simulink model "FFR_3area_2"  (R2015a)
settings: Solver=ode45  StartTime=0.0  StopTime=100  RelTol=1e-3
values from neighbouring files (symbols this model uses):
  beta = [0.3483 0.3827 0.3692]    [init_FFR_3area.m]    (also in init_FFR_3area_2.m; init_FFR_3area_3.m; init_FFR_3area_4.m; init_FFR_3area_5.m)
  D = 0.015    [init_FFR_1_0.m]    (also in init_FFR_1_1.m; init_FFR_3area.m = [0.015 0.016 0.015]; init_FFR_3area_2.m = [0.015 0.016 0.015]; init_FFR_3area_3.m = [0.015 0.016 0.015])
  H = 0.0833    [init_FFR_1_0.m]    (also in init_FFR_1_1.m; init_FFR_3area.m = [0.1667 0.2017 0.1247] .* 0.5; init_FFR_3area_2.m = [0.1667 0.2017 0.1247] .* 0.5; init_FFR_3area_3.m = [0.1667 0.2017 0.1247] .* 0.5)
  Ki = -0.3    [init_FFR_1_0.m]    (also in init_FFR_1_1.m = -2; init_FFR_3area.m = [-0.3 -0.2 -0.4]; init_FFR_3area_2.m = [-0.3 -0.2 -0.4]; init_FFR_3area_3.m = [-0.3 -0.2 -0.4])
  R = 3    [init_FFR_1_0.m]    (also in init_FFR_1_1.m; init_FFR_3area.m = [3 2.73 2.82]; init_FFR_3area_2.m = [3 2.73 2.82]; init_FFR_3area_3.m = [3 2.73 2.82])
  T_12 = 0.20    (= 0.2)    [allocateProduction.m]    (also in allocation.m; init_FFR_3area.m; init_FFR_3area_2.m; init_FFR_3area_3.m)
  T_13 = 0.25    [allocateProduction.m]    (also in allocation.m; init_FFR_3area.m; init_FFR_3area_2.m; init_FFR_3area_3.m)
  T_21 = 0.20    (= 0.2)    [allocateProduction.m]    (also in allocation.m; init_FFR_3area.m; init_FFR_3area_2.m; init_FFR_3area_3.m)
  T_23 = 0.12    [allocateProduction.m]    (also in allocation.m; init_FFR_3area.m; init_FFR_3area_2.m; init_FFR_3area_3.m)
  T_31 = 0.25    [allocateProduction.m]    (also in allocation.m; init_FFR_3area.m; init_FFR_3area_2.m; init_FFR_3area_3.m)
  T_32 = 0.12    [allocateProduction.m]    (also in allocation.m; init_FFR_3area.m; init_FFR_3area_2.m; init_FFR_3area_3.m)
  T_g = 0.08    [init_FFR_1_0.m]    (also in init_FFR_1_1.m; init_FFR_3area.m = [0.08 0.06 0.07]; init_FFR_3area_2.m = [0.08 0.06 0.07]; init_FFR_3area_3.m = [0.08 0.06 0.07])
  T_t = 0.40    (= 0.4)    [init_FFR_1_0.m]    (also in init_FFR_1_1.m; init_FFR_3area.m = [0.40 0.44 0.30]; init_FFR_3area_2.m = [0.40 0.44 0.30]; init_FFR_3area_3.m = [0.40 0.44 0.30])
libraries: simulink x3, aerolibanimutils x1
settings Model: Creator=tarje  LastModifiedBy=tarje

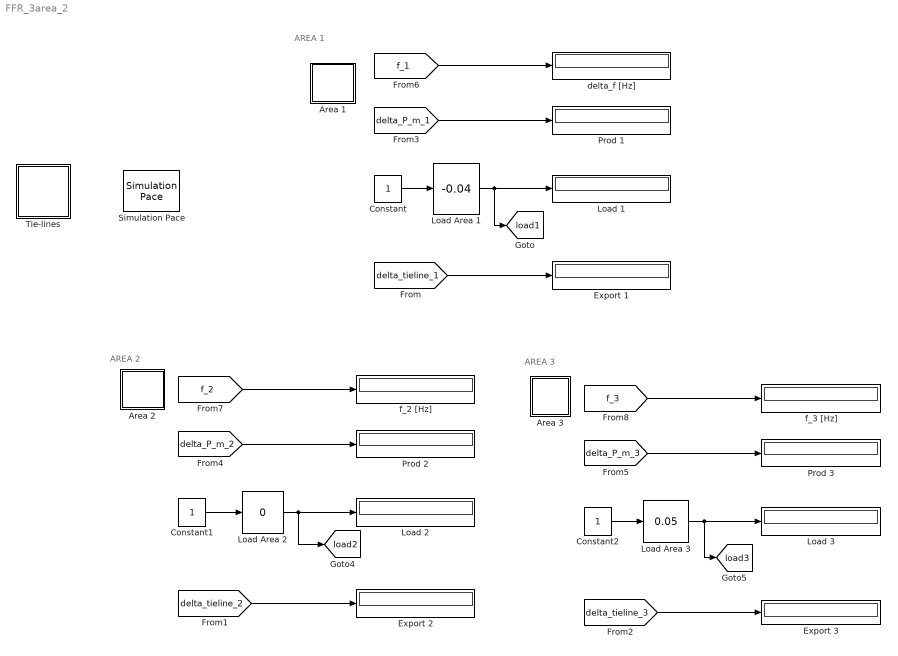
== system FFR_3area_2 ==
  note: AREA 3
  note: AREA 2
  note: AREA 1
  Area 1 : Subsystem
  Area 2 : Subsystem
  Area 3 : Subsystem
  Constant : Constant
  Constant1 : Constant
  Constant2 : Constant
  Export 1 : Display
  Export 2 : Display
  Export 3 : Display
  Load 1 : Display
  Load 2 : Display
  Load 3 : Display
  Load Area 1 : simulink/Math Operations/Slider Gain  low=-0.2  gain=-0.04  high=0.2
  Load Area 2 : simulink/Math Operations/Slider Gain  low=-0.05  gain=0  high=1
  Load Area 3 : simulink/Math Operations/Slider Gain  low=-0.05  gain=0.05  high=0.05
  Prod 1 : Display
  Prod 2 : Display
  Prod 3 : Display
  Simulation Pace : aerolibanimutils/Simulation Pace  SimulationPace=1  SleepMode=MATLAB Thread  OutputPaceError=off  SampleTime=1/30
      settings: AttributesFormatString=%<SimulationPace> sec/sec
  Tie-lines : Subsystem
  delta_f [Hz] : Display
  f_2 [Hz] : Display
  f_3 [Hz] : Display
  tag scope: load1=global, load2=global, load3=global
  wires:
  [f_1] -> delta_f [Hz]/1
  [delta_P_m_1] -> Prod 1/1
  Constant/1 -> Load Area 1/1
  Load Area 1/1 -> [load1], Load 1/1
  [f_2] -> f_2 [Hz]/1
  [delta_P_m_2] -> Prod 2/1
  Constant1/1 -> Load Area 2/1
  Load Area 2/1 -> [load2], Load 2/1
  [f_3] -> f_3 [Hz]/1
  [delta_P_m_3] -> Prod 3/1
  Constant2/1 -> Load Area 3/1
  Load Area 3/1 -> [load3], Load 3/1
  [delta_tieline_1] -> Export 1/1
  [delta_tieline_2] -> Export 2/1
  [delta_tieline_3] -> Export 3/1

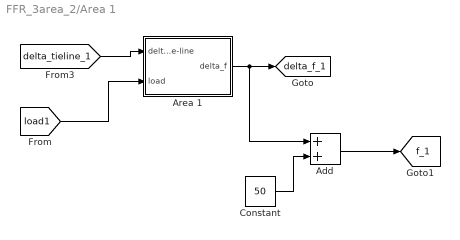
== system FFR_3area_2/Area 1 ==
  Add : Sum
  Area 1 : Subsystem
  Constant : Constant  Value=50
  tag scope: delta_f_1=global, f_1=global
  wires:
  [delta_tieline_1] -> Area 1/1(delta_tie-line)
  Area 1/1(delta_f) -> Add/1, [delta_f_1]
  [load1] -> Area 1/2(load)
  Constant/1 -> Add/2
  Add/1 -> [f_1]

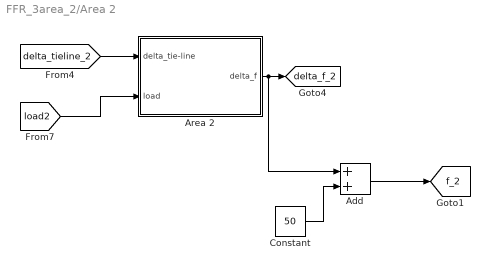
== system FFR_3area_2/Area 2 ==
  Add : Sum
  Area 2 : Subsystem
  Constant : Constant  Value=50
  tag scope: delta_f_2=global, f_2=global
  wires:
  Area 2/1(delta_f) -> Add/1, [delta_f_2]
  [load2] -> Area 2/2(load)
  [delta_tieline_2] -> Area 2/1(delta_tie-line)
  Constant/1 -> Add/2
  Add/1 -> [f_2]

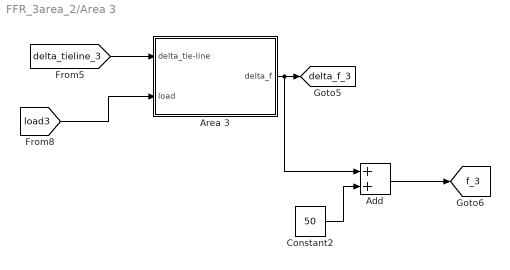
== system FFR_3area_2/Area 3 ==
  Add : Sum
  Area 3 : Subsystem
  Constant2 : Constant  Value=50
  tag scope: delta_f_3=global, f_3=global
  wires:
  [load3] -> Area 3/2(load)
  Area 3/1(delta_f) -> Add/1, [delta_f_3]
  [delta_tieline_3] -> Area 3/1(delta_tie-line)
  Add/1 -> [f_3]
  Constant2/1 -> Add/2

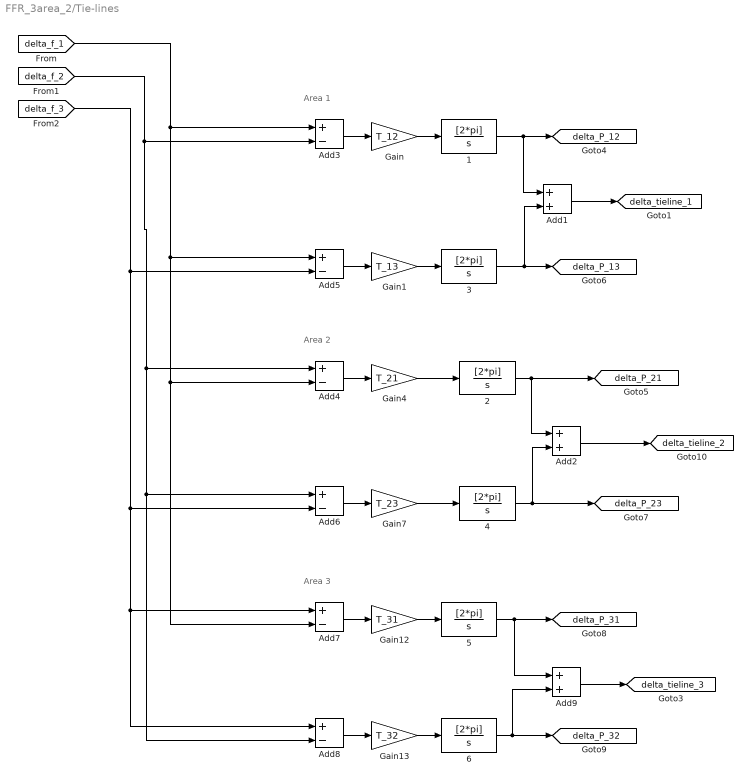
== system FFR_3area_2/Tie-lines ==
  note: Area 3
  note: Area 2
  note: Area 1
   {1..6} (6 alike) : TransferFcn  Numerator=[2*pi]  Denominator=[1 0]
  Add1 : Sum
  Add2 : Sum
  Add{3..8} (6 alike) : Sum  Inputs=+-
  Add9 : Sum
  Gain : Gain  Gain=T_12
  Gain1 : Gain  Gain=T_13
  Gain12 : Gain  Gain=T_31
  Gain13 : Gain  Gain=T_32
  Gain4 : Gain  Gain=T_21
  Gain7 : Gain  Gain=T_23
  tag scope: delta_P_12=global, delta_P_13=global, delta_P_21=global, delta_P_23=global, delta_P_31=global, delta_P_32=global, delta_tieline_1=global, delta_tieline_2=global, delta_tieline_3=global
  wires:
  [delta_f_2] -> Add3/2, Add8/2, Add6/1, Add4/1
  [delta_f_1] -> Add3/1, Add5/1, Add7/2, Add4/2
  [delta_f_3] -> Add5/2, Add8/1, Add7/1, Add6/2
  " 1"/1 -> Add1/1, [delta_P_12]
  Add3/1 -> Gain/1
  " 2"/1 -> Add2/1, [delta_P_21]
  Add4/1 -> Gain4/1
  " 3"/1 -> Add1/2, [delta_P_13]
  Add5/1 -> Gain1/1
  " 4"/1 -> Add2/2, [delta_P_23]
  Add6/1 -> Gain7/1
  " 5"/1 -> Add9/1, [delta_P_31]
  Add7/1 -> Gain12/1
  " 6"/1 -> Add9/2, [delta_P_32]
  Add8/1 -> Gain13/1
  Add9/1 -> [delta_tieline_3]
  Gain12/1 -> " 5"/1
  Gain13/1 -> " 6"/1
  Add2/1 -> [delta_tieline_2]
  Gain4/1 -> " 2"/1
  Gain7/1 -> " 4"/1
  Add1/1 -> [delta_tieline_1]
  Gain/1 -> " 1"/1
  Gain1/1 -> " 3"/1

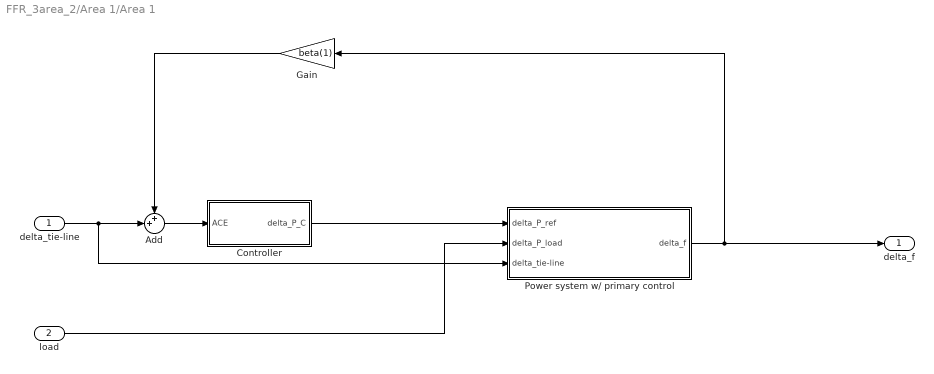
== system FFR_3area_2/Area 1/Area 1 ==
  delta_tie-line : Inport
  load : Inport  Port=2
  Add : Sum  Inputs=++|
  Controller : Subsystem
  Gain : Gain  Gain=beta(1)
  Power system w/ primary control : Subsystem
  delta_f : Outport
  wires:
  Controller/1(delta_P_C) -> Power system w/ primary control/1(delta_P_ref)
  Power system w/ primary control/1(delta_f) -> Gain/1, delta_f/1
  Gain/1 -> Add/1
  delta_tie-line/1 -> Power system w/ primary control/3(delta_tie-line), Add/2
  Add/1 -> Controller/1(ACE)
  load/1 -> Power system w/ primary control/2(delta_P_load)

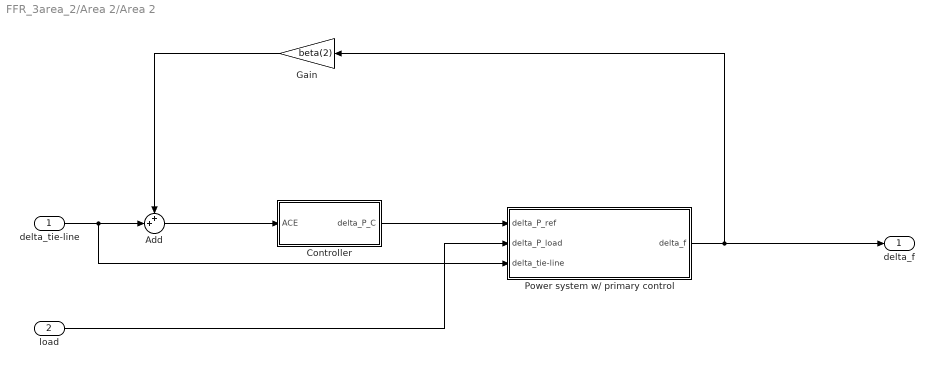
== system FFR_3area_2/Area 2/Area 2 ==
  delta_tie-line : Inport
  load : Inport  Port=2
  Add : Sum  Inputs=++|
  Controller : Subsystem
  Gain : Gain  Gain=beta(2)
  Power system w/ primary control : Subsystem
  delta_f : Outport
  wires:
  Controller/1(delta_P_C) -> Power system w/ primary control/1(delta_P_ref)
  Power system w/ primary control/1(delta_f) -> Gain/1, delta_f/1
  Gain/1 -> Add/1
  delta_tie-line/1 -> Power system w/ primary control/3(delta_tie-line), Add/2
  Add/1 -> Controller/1(ACE)
  load/1 -> Power system w/ primary control/2(delta_P_load)

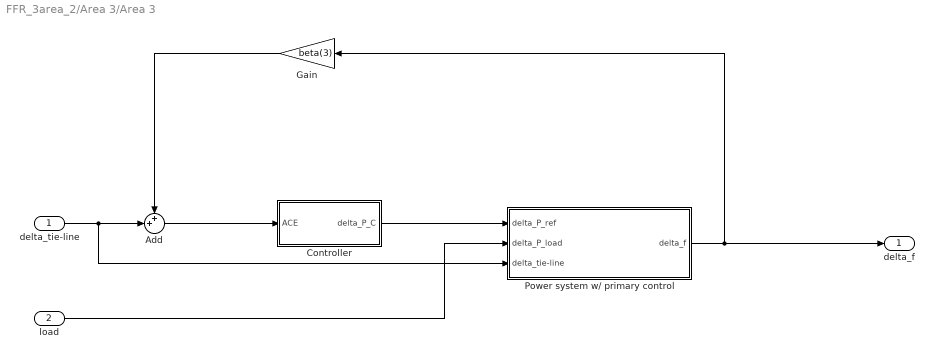
== system FFR_3area_2/Area 3/Area 3 ==
  delta_tie-line : Inport
  load : Inport  Port=2
  Add : Sum  Inputs=++|
  Controller : Subsystem
  Gain : Gain  Gain=beta(3)
  Power system w/ primary control : Subsystem
  delta_f : Outport
  wires:
  Controller/1(delta_P_C) -> Power system w/ primary control/1(delta_P_ref)
  Power system w/ primary control/1(delta_f) -> Gain/1, delta_f/1
  Gain/1 -> Add/1
  delta_tie-line/1 -> Power system w/ primary control/3(delta_tie-line), Add/2
  Add/1 -> Controller/1(ACE)
  load/1 -> Power system w/ primary control/2(delta_P_load)

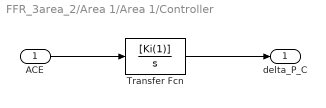
== system FFR_3area_2/Area 1/Area 1/Controller ==
  ACE : Inport
  Transfer Fcn : TransferFcn  Numerator=[Ki(1)]  Denominator=[1 0]
  delta_P_C : Outport
  wires:
  ACE/1 -> Transfer Fcn/1
  Transfer Fcn/1 -> delta_P_C/1

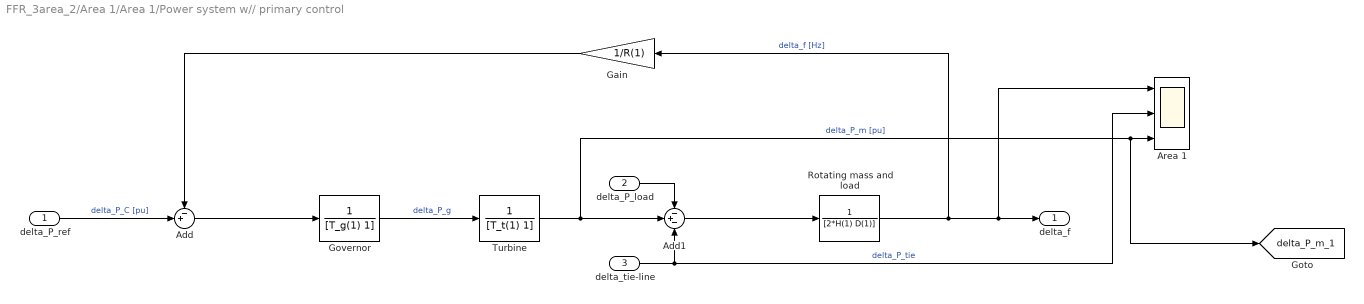
== system FFR_3area_2/Area 1/Area 1/Power system w// primary control ==
  delta_P_ref : Inport
  delta_P_load : Inport  Port=2
  delta_tie-line : Inport  Port=3
  Add : Sum  Inputs=-+|
  Add1 : Sum  Inputs=-+-
  Area 1 : Scope  NumInputPorts=3
      settings: TimeRange=3.2  YMin=-0.06~-0.02~-0.01  YMax=0.1~0.025~0.03
  Gain : Gain  Gain=1/R(1)
  Governor : TransferFcn  Denominator=[T_g(1) 1]
  Rotating mass and load : TransferFcn  Denominator=[2*H(1) D(1)]
  Turbine : TransferFcn  Denominator=[T_t(1) 1]
  delta_f : Outport
  tag scope: delta_P_m_1=global
  wires:
  Turbine/1 -> [delta_P_m_1], Area 1/3, Add1/2  "delta_P_m [pu]"
  Rotating mass and load/1 -> Area 1/1, delta_f/1, Gain/1  "delta_f [Hz]"
  Gain/1 -> Add/1
  Add1/1 -> Rotating mass and load/1
  Add/1 -> Governor/1
  Governor/1 -> Turbine/1  "delta_P_g"
  delta_P_ref/1 -> Add/2  "delta_P_C [pu]"
  delta_P_load/1 -> Add1/1
  delta_tie-line/1 -> Area 1/2, Add1/3  "delta_P_tie"

== system FFR_3area_2/Area 2/Area 2/Controller ==
  ACE : Inport
  Transfer Fcn : TransferFcn  Numerator=[Ki(2)]  Denominator=[1 0]
  delta_P_C : Outport
  wires:
  ACE/1 -> Transfer Fcn/1
  Transfer Fcn/1 -> delta_P_C/1

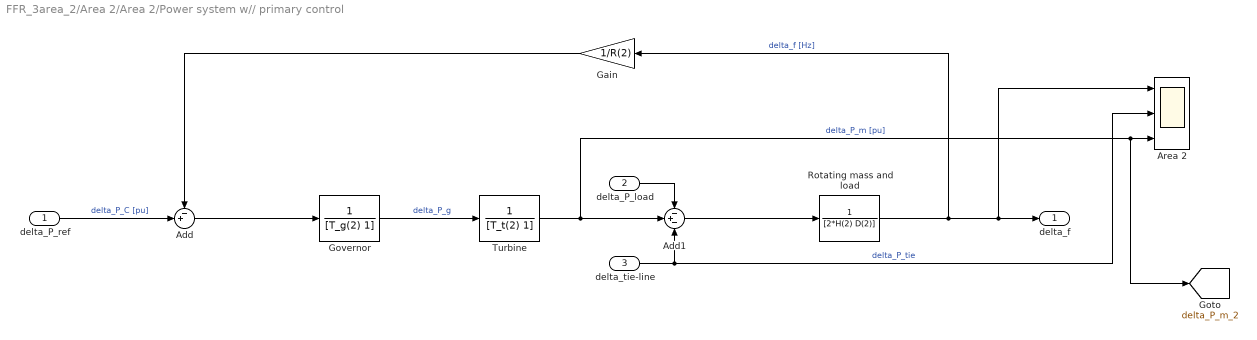
== system FFR_3area_2/Area 2/Area 2/Power system w// primary control ==
  delta_P_ref : Inport
  delta_P_load : Inport  Port=2
  delta_tie-line : Inport  Port=3
  Add : Sum  Inputs=-+|
  Add1 : Sum  Inputs=-+-
  Area 2 : Scope  NumInputPorts=3
      settings: TimeRange=15  YMin=-0.08~-0.005~-0.01  YMax=0.025~0.04~0.03
  Gain : Gain  Gain=1/R(2)
  Governor : TransferFcn  Denominator=[T_g(2) 1]
  Rotating mass and load : TransferFcn  Denominator=[2*H(2) D(2)]
  Turbine : TransferFcn  Denominator=[T_t(2) 1]
  delta_f : Outport
  tag scope: delta_P_m_2=global
  wires:
  Turbine/1 -> [delta_P_m_2], Area 2/3, Add1/2  "delta_P_m [pu]"
  Rotating mass and load/1 -> Area 2/1, delta_f/1, Gain/1  "delta_f [Hz]"
  Gain/1 -> Add/1
  Add1/1 -> Rotating mass and load/1
  Add/1 -> Governor/1
  Governor/1 -> Turbine/1  "delta_P_g"
  delta_P_ref/1 -> Add/2  "delta_P_C [pu]"
  delta_P_load/1 -> Add1/1
  delta_tie-line/1 -> Area 2/2, Add1/3  "delta_P_tie"

== system FFR_3area_2/Area 3/Area 3/Controller ==
  ACE : Inport
  Transfer Fcn : TransferFcn  Numerator=[Ki(3)]  Denominator=[1 0]
  delta_P_C : Outport
  wires:
  ACE/1 -> Transfer Fcn/1
  Transfer Fcn/1 -> delta_P_C/1

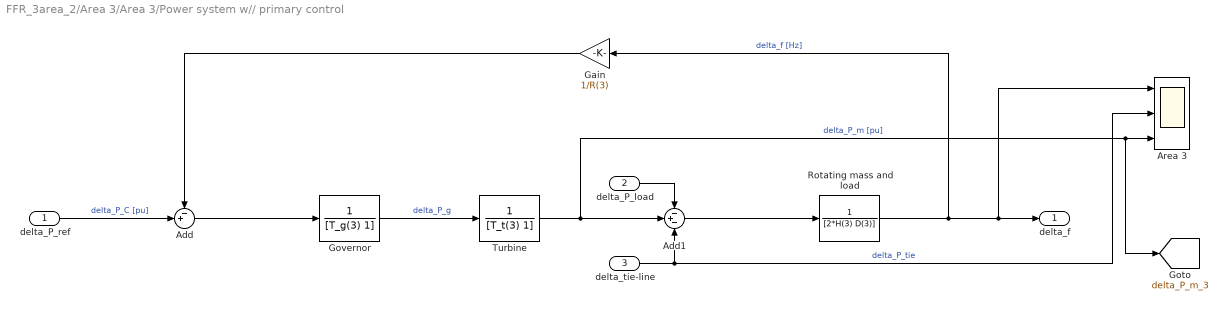
== system FFR_3area_2/Area 3/Area 3/Power system w// primary control ==
  delta_P_ref : Inport
  delta_P_load : Inport  Port=2
  delta_tie-line : Inport  Port=3
  Add : Sum  Inputs=-+|
  Add1 : Sum  Inputs=-+-
  Area 3 : Scope  NumInputPorts=3
      settings: TimeRange=15  YMin=-0.08~-0.005~-0.01  YMax=0.025~0.04~0.03
  Gain : Gain  Gain=1/R(3)
  Governor : TransferFcn  Denominator=[T_g(3) 1]
  Rotating mass and load : TransferFcn  Denominator=[2*H(3) D(3)]
  Turbine : TransferFcn  Denominator=[T_t(3) 1]
  delta_f : Outport
  tag scope: delta_P_m_3=global
  wires:
  Turbine/1 -> [delta_P_m_3], Area 3/3, Add1/2  "delta_P_m [pu]"
  Rotating mass and load/1 -> Area 3/1, delta_f/1, Gain/1  "delta_f [Hz]"
  Gain/1 -> Add/1
  Add1/1 -> Rotating mass and load/1
  Add/1 -> Governor/1
  Governor/1 -> Turbine/1  "delta_P_g"
  delta_P_ref/1 -> Add/2  "delta_P_C [pu]"
  delta_P_load/1 -> Add1/1
  delta_tie-line/1 -> Area 3/2, Add1/3  "delta_P_tie"
